simulink model "tracking_controller"  (R2015a)
settings: Solver=FixedStepDiscrete  StartTime=0.0  StopTime=inf  FixedStep=sample_time  RelTol=1e-3
StartFcn:
  | tg.sampletime = correctedSampleTime;
libraries: slrtlib x1
settings Model: SimulationMode=external  ParamWorkspaceSource=ReferencedWorkspace  CovSFcnEnable=off  Creator=wmartin  LastModifiedBy=robots
settings SolverCC: EnableConcurrentExecution=on
settings DataIOCC: LimitDataPoints=off  MaxDataPoints=1e7  SaveFormat=StructureWithTime  SignalLogging=off  DSMLogging=off
settings OptimizationCC: BlockReduction=off  OptimizeBlockIOStorage=off  BufferReuse=off  GlobalBufferReuse=off  ExpressionFolding=off  ExpressionDepthLimit=2147483647  LocalBlockOutputs=off  SimCompilerOptimization=on
settings DebuggingCC: UnderspecifiedInitializationDetection=Classic  MergeDetectMultiDrivingBlocksExec=none  SolverPrmCheckMsg=warning  StateNameClashWarn=warning
settings HardwareCC: ProdIntDivRoundTo=Zero  ProdEndianess=LittleEndian  ProdLongLongMode=on  ProdHWDeviceType=Generic->32-bit x86 compatible
settings ModelReferenceCC: UpdateModelReferenceTargets=IfOutOfDate  ModelReferenceNumInstancesAllowed=Single  ModelReferenceMinAlgLoopOccurrences=on
settings RTWCC: SystemTargetFile=slrt.tlc  TemplateMakefile=slrt_default_tmf  Description=Simulink Real-Time  RTWVerbose=off  RTWCompilerOptimization=on
settings CodeAppCC: MaxIdLength=256
settings SimulinkRealTimeCC: GeneratePreprocessorConditionals=Disable all  RL32LogBufSizeModifier=1e8

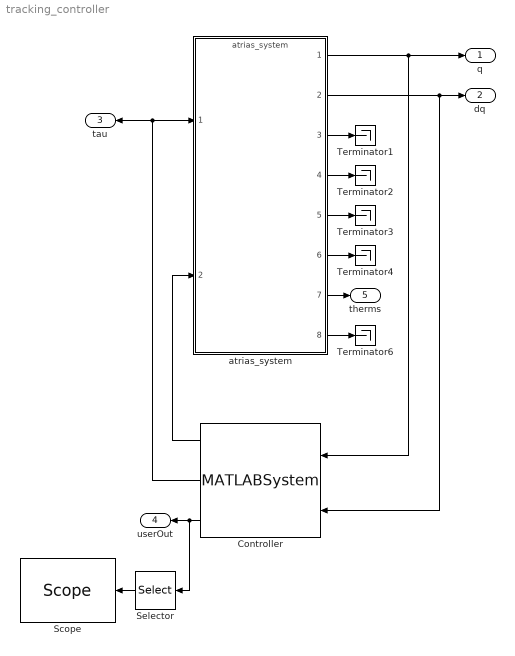
== system tracking_controller ==
  Controller : MATLABSystem  System=TrackingController  kp_leg=4000  kd_leg=150  s_l_A=0.9  s_l_B=1.17  s_r_A=1.08  s_r_B=1.13  kp_hip=2000  kd_hip=75  l_A=0.1  q_A=0.2  f_c=0  f_v=0  isSim=off  ps3Axes=[0 0 0 0]  ps3Buttons=[0 0 0 0 0 0 0 0 0 0 0 0 0 0 0 0 0]  u_lim=714  SimulateUsing=Code generation
      mask Type: TrackingController
      mask Display:
      | disp('TrackingController');
      | port_label('input',1,'q');
      | port_label('input',2,'dq');
      | port_label('output',1,'eStop');
      | port_label('output',2,'u');
      | port_label('output',3,'userOut');
  "Scope " : slrtlib/Displays and Logging/Scope   scopeno=1  scopetype=Host  autostart=on  viewmode=Graphical redraw  formatstr='%15.6f'  grid=on  ylimits=[0,0]  nosamples=1000  noprepostsamples=0  interleave=1  triggermode=FreeRun  triggersignal=1  trigsignalfromport=off  triggerlevel=0.0  triggerslope=Either  triggerscope=1  triggersample=0  filename=data.dat  mode=Lazy  writesize=512  autorestart=off  dynamicfilemode=off  maxwritefilesize=512*1024^2
  Selector : Selector  InputPortWidth=8  Indices=[1:4]
  Terminator{1..4,6} (5 alike) : Terminator
  atrias_system : ModelReference  ModelNameDialog=atrias_system  SimulationMode=Normal  ModelReferenceVersion=1.2773  CopyOfModelName=atrias_system  DefaultDataLogging=on
  q : Outport
  dq : Outport  Port=2
  tau : Outport  Port=3
  userOut : Outport  Port=4
  therms : Outport  Port=5
  wires:
  atrias_system/2 -> Controller/2, dq/1
  atrias_system/1 -> Controller/1, q/1
  atrias_system/3 -> Terminator1/1
  atrias_system/6 -> Terminator4/1
  atrias_system/5 -> Terminator3/1
  atrias_system/7 -> therms/1
  Controller/2 -> atrias_system/1, tau/1
  Controller/1 -> atrias_system/2
  atrias_system/8 -> Terminator6/1
  Controller/3 -> Selector/1, userOut/1
  Selector/1 -> "Scope "/1
  atrias_system/4 -> Terminator2/1
